simulink model "reverse_pendulum"  (R2021b)
settings: Solver=VariableStepAuto  StartTime=0.0  StopTime=30  MaxStep=0.05  RelTol=1e-3
libraries: simulink_extras x1, slpidlib x1
settings Model: Creator=user  LastModifiedBy=user

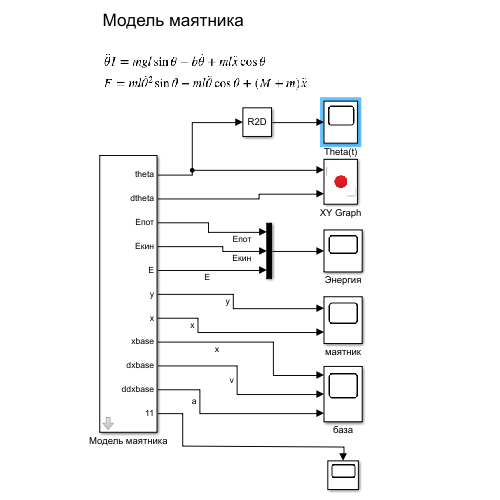
[thumbnail: Simulink's stored preview of the top-level diagram]
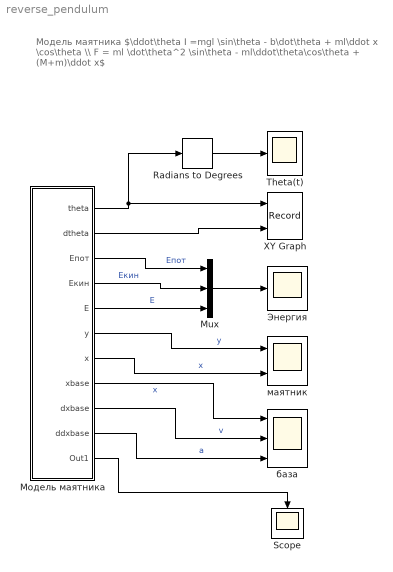
== system reverse_pendulum ==
  note: Модель маятника
      |
      | $\ddot\theta I =mgl \sin\theta - b\dot\theta + ml\ddot x \cos\theta \\ F = ml \dot\theta^2 \sin\theta - ml\ddot\theta\cos\theta + (M+m)\ddot x$
  Mux : Mux  Inputs=3
  Radians to Degrees : simulink_extras/Transformations/Radians to Degrees
  Scope : Scope
  Theta(t) : Scope
  XY Graph : Record  FileSettingsInternal="{\"entries\":[{\"content\":{\"excelSettings\":{\"content\":{},\"type\":\"Streamout.ExcelSettings\"}},\"type\":\"Streamout.FileSettingStorage\",\"uuid\":\"0c6cba2f-ecbe-4051-b816-abee11555979\"}],\"packageUris\":[\"http://schema.mathworks.com/mf0/streamout_blocks/R2020a\"],\"version\":\"1.0\"}"  Layout=[1 1]  SignalsInternal="{\"entries\":[{\"content\":{\"signals\":[{\"content\":{\"blockPath\":[\"reverse_pendulum/XY Graph\"],\"channel\":[],\"dimensions\":[1],\"domain\":\"reverse_pendulum/XY Graph\",\"lineColor\":\"#a2142f\",\"plots\":[1],\"port\":1,\"sid\":[\"\"],\"signalID\":59,\"signalName\":\"Модель маятника:1\"},\"type\":\"RecordBlkView.Signal\",\"uuid\":\"2ba1622c-7781-4ceb-bd01-50b734ef610a\"},{\"content\":{\"blockPath\":[\"reverse_pendulum/XY Graph\"],\"channel\":[],\"dimensions\":[1],\"domain\":\"reverse_pendulum/XY Graph\",\"lineColor\":\"#139fff\",\"plots\":[1],\"port\":2,\"sid\":[\"\"],\"signalID\":63,\"signalName\":\"Модель маятника:2\"},\"type\":\"RecordBlkView.Signal\",\"uuid\":\"4942546b-33a2-4686-bbd8-b75294cda65a\"}]},\"type\":\"RecordBlkView.InputSignals\",\"uuid\":\"2b6629fe-66d5-4971-8b58-ddfc7d3b512e\"}],\"packageUris\":[\"http://schema.mathworks.com/mf0/streamout_blocks/R2020a\"],\"version\":\"1.0\"}"  VisualizationBindings="{\"xyplotplugin\":{\"info\":[{\"series\":[{\"bindingParametersList\":[{\"parameter\":\"X-Axis\",\"signalID\":59,\"signalName\":\"РњРѕРґРµР»СЊ РјР°СЏС‚РЅРёРєР°:1\"},{\"parameter\":\"Y-Axis\",\"signalID\":63,\"signalName\":\"РњРѕРґРµР»СЊ РјР°СЏС‚РЅРёРєР°:2\"}],\"seriesID\":10508}],\"subplotID\":1}]}}"  CompatibilityTag=XY
  Модель маятника : Subsystem  mask{m=1, l=1, g=9.8, startDegree=30, b=0, Mp=10, F=0}
      mask prompts: m "масса"; l "длина подвеса"; g "ускорение свободного падения"; startDegree "стартовый угол"; b "диссипативный член"; Mp "масса платформы"; F "сила"
      mask init:
      | I = m * l^2
  Энергия : Scope
  база : Scope  NumInputPorts=3
  маятник : Scope  NumInputPorts=2
  wires:
  Модель маятника/7(x) -> маятник/2  "x"
  Модель маятника/2(dtheta) -> XY Graph/2
  Radians to Degrees/1 -> Theta(t)/1
  Mux/1 -> Энергия/1
  Модель маятника/5(Е) -> Mux/3  "E"
  Модель маятника/1(theta) -> Radians to Degrees/1, XY Graph/1
  Модель маятника/3(Eпот) -> Mux/1  "Eпот"
  Модель маятника/6(y) -> маятник/1  "y"
  Модель маятника/4(Екин) -> Mux/2  "Екин"
  Модель маятника/8(xbase) -> база/1  "x"
  Модель маятника/9(dxbase) -> база/2  "v"
  Модель маятника/10(ddxbase) -> база/3  "a"
  Модель маятника/11(Out1) -> Scope/1

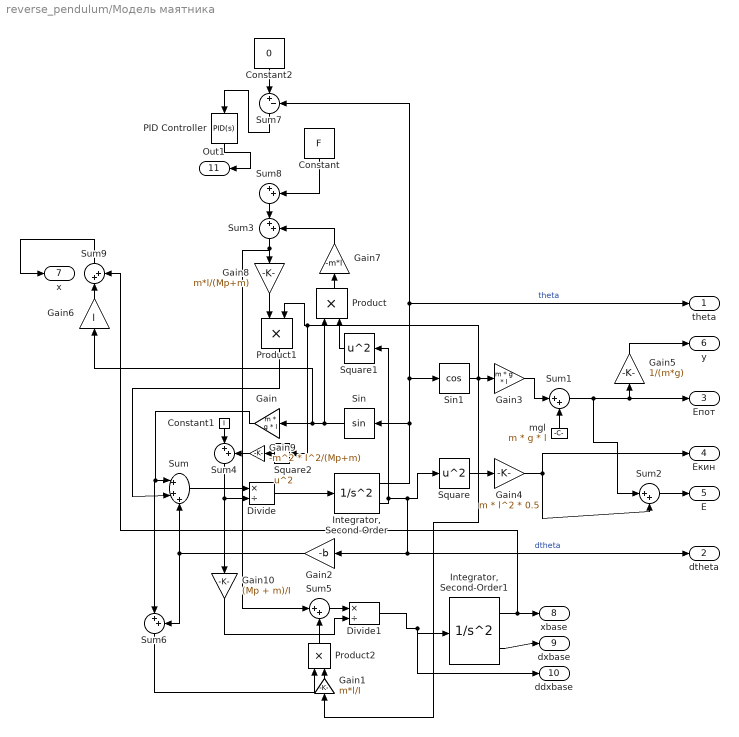
== system reverse_pendulum/Модель маятника ==
  Constant : Constant  Value=F
  Constant1 : Constant  Value=I
  Constant2 : Constant  Value=0
  Divide : Product  Inputs=*/
  Divide1 : Product  Inputs=*/
  Gain : Gain  Gain=m * g * l
  Gain1 : Gain  Gain=m*l/I
  Gain10 : Gain  Gain=(Mp + m)/I
  Gain2 : Gain  Gain=-b
  Gain3 : Gain  Gain=m * g * l
  Gain4 : Gain  Gain=m * l^2 * 0.5
  Gain5 : Gain  Gain=1/(m*g)
  Gain6 : Gain  Gain=l
  Gain7 : Gain  Gain=-m*l
  Gain8 : Gain  Gain=m*l/(Mp+m)
  Gain9 : Gain  Gain=-m^2 * l^2/(Mp+m)
  "Integrator, Second-Order" : SecondOrderIntegrator  ICX=deg2rad(startDegree)
  "Integrator, Second-Order1" : SecondOrderIntegrator
  PID Controller : slpidlib/PID Controller  Controller=PID  Form=Parallel  TimeDomain=Continuous-time  UseExternalTs=off  SampleTime=-1  IntegratorMethod=Forward Euler  FilterMethod=Forward Euler  ControllerParametersSource=internal  P=150  I=0  D=35  UseFilter=on  N=100  TunerSelectOption=Transfer Function Based (PID Tuner App)  InitialConditionSource=internal  InitialConditionForIntegrator=0  InitialConditionForFilter=0  DifferentiatorICPrevScaledInput=0  ExternalReset=none  TrackingMode=off  Kt=1  LimitOutput=off  SatLimitsSource=internal  UpperSaturationLimit=inf  LowerSaturationLimit=-inf  LinearizeAsGain=on  AntiWindupMode=none  Kb=1  POutMin=[]  POutMax=[]  IOutMin=[]  IOutMax=[]  DOutMin=[]  DOutMax=[]  NOutMin=[]  NOutMax=[]  SumOutMin=[]  SumOutMax=[]  SaturationOutMin=[]  SaturationOutMax=[]  PParamMin=[]  PParamMax=[]  IParamMin=[]  IParamMax=[]  DParamMin=[]  DParamMax=[]  NParamMin=[]  NParamMax=[]  KbParamMin=[]  KbParamMax=[]  KtParamMin=[]  KtParamMax=[]  KbOutMin=[]  KbOutMax=[]  KtOutMin=[]  KtOutMax=[]  IntegratorOutMin=[]  IntegratorOutMax=[]  FilterOutMin=[]  FilterOutMax=[]  SumI1OutMin=[]  SumI1OutMax=[]  SumI2OutMin=[]  SumI2OutMax=[]  SumI3OutMin=[]  SumI3OutMax=[]  SumI4OutMin=[]  SumI4OutMax=[]  SumDOutMin=[]  SumDOutMax=[]  DifferentiatorOutMin=[]  DifferentiatorOutMax=[]  FilterDiffOutCoefMin=[]  FilterDiffOutCoefMax=[]  ReciprocalOutMin=[]  ReciprocalOutMax=[]  SumDenOutMin=[]  SumDenOutMax=[]  SumNumOutMin=[]  SumNumOutMax=[]  DivideOutMin=[]  DivideOutMax=[]  UdiffTsProdOutMin=[]  UdiffTsProdOutMax=[]  NTsProdOutMin=[]  NTsProdOutMax=[]  UintegralTsProdOutMin=[]  UintegralTsProdOutMax=[]  UngainTsProdOutMin=[]  UngainTsProdOutMax=[]  IntegratorContinuousStateAttributes=''  IntegratorStateMustResolveToSignalObject=off  IntegratorRTWStateStorageClass=Auto  FilterContinuousStateAttributes=''  FilterStateMustResolveToSignalObject=off  FilterRTWStateStorageClass=Auto  ParallelPVariant=InternalParameters  IdealPVariant=Disabled  IVariant=InternalParameters  DVariant=InternalParameters  IntegratorVariant=Continuous  SatVariant=Disabled  AWVariant=Passthrough  PCopyVariant=Disabled  TRVariant=Disabled  FdbkBlocksVariant=Forward  IdealPFdbkVariant=Disabled  SatFdbkVariant=Disabled  DerivativeFilterVariant=ContFilter  NVariant=InternalParameters  NCopyVariant=Disabled  FilterICVariant=InternalICsFilter  IntegratorICVariant=InternalICs  ExternalResetVariant=Disabled  TRSumVariant=Passthrough  SumFdbkVariant=Disabled  SumVariant=Sum_PID  TsampFilterVariant=InternalTs  TsampNgainVariant=Passthrough  TsampIntegralVariant=Passthrough  ExternalSaturationOutDataTypeStr=Inherit: Same as second input
  Product : Product
  Product1 : Product
  Product2 : Product
  Sin : Trigonometry
  Sin1 : Trigonometry  Operator=cos
  Square : Math  Operator=square  SaturateOnIntegerOverflow=on
  Square1 : Math  Operator=square  SaturateOnIntegerOverflow=on
  Square2 : Math  Operator=square  SaturateOnIntegerOverflow=on
  Sum : Sum  Inputs=|+++
  Sum{1..6,8..9} (8 alike) : Sum  Inputs=|++
  Sum7 : Sum  Inputs=|+-
  mgl : Constant  Value=m * g * l
  theta : Outport
  dtheta : Outport  Port=2
  Eпот : Outport  Port=3
  Екин : Outport  Port=4
  Е : Outport  Port=5
  y : Outport  Port=6
  x : Outport  Port=7
  xbase : Outport  Port=8
  dxbase : Outport  Port=9
  ddxbase : Outport  Port=10
  Out1 : Outport  Port=11
  wires:
  Sin/1 -> Gain/1, Gain6/1, Product/1
  "Integrator, Second-Order"/1 -> Sin1/1, Sum7/2, theta/1, Sin/1  "theta"
  "Integrator, Second-Order"/2 -> Square1/1, Gain2/1, dtheta/1, Square/1  "dtheta"
  Sin1/1 -> Gain1/1, Square2/1, Product1/2, Gain3/1
  mgl/1 -> Sum1/2
  Gain3/1 -> Sum1/1
  Square/1 -> Gain4/1
  Gain4/1 -> Sum2/2, Екин/1
  Sum2/1 -> Е/1
  Sum1/1 -> Sum2/1, Gain5/1, Eпот/1
  Gain5/1 -> y/1
  Square1/1 -> Product/2
  Product/1 -> Gain7/1
  Gain7/1 -> Sum3/2
  Sum3/1 -> Sum5/1, Gain8/1
  Gain8/1 -> Product1/1
  Gain2/1 -> Sum6/2, Sum/3
  Gain/1 -> Sum6/1, Sum/1
  Product1/1 -> Sum/2
  Square2/1 -> Gain9/1
  Gain9/1 -> Sum4/2
  Constant1/1 -> Sum4/1
  Sum/1 -> Divide/1
  Divide/1 -> "Integrator, Second-Order"/1
  Sum4/1 -> Gain10/1, Divide/2
  Gain1/1 -> Product2/2
  Product2/1 -> Sum5/2
  Sum6/1 -> Product2/1
  Sum5/1 -> Divide1/1
  Gain10/1 -> Divide1/2
  Divide1/1 -> ddxbase/1, "Integrator, Second-Order1"/1
  "Integrator, Second-Order1"/2 -> dxbase/1
  "Integrator, Second-Order1"/1 -> Sum9/2, xbase/1
  Sum7/1 -> PID Controller/1
  Constant2/1 -> Sum7/1
  PID Controller/1 -> Out1/1
  Constant/1 -> Sum8/2
  Sum8/1 -> Sum3/1
  Gain6/1 -> Sum9/1
  Sum9/1 -> x/1
